simulink model "Model"  (R2016a)
settings: Solver=ode23tb  StartTime=0.0  StopTime=1  RelTol=1e-3
libraries: powerlib_meascontrol x6, powerlib x6
settings Model: Creator=Rodney Tan  LastModifiedBy=Rodney Tan
settings DataIOCC: LimitDataPoints=on  SaveFormat=Array
settings DebuggingCC: SolverPrmCheckMsg=warning
settings HardwareCC: ProdBitPerPointer=32  ProdLargestAtomicFloat=None  ProdIntDivRoundTo=Undefined  ProdEndianess=Unspecified  ProdWordSize=32  ProdHWDeviceType=32-bit Generic
settings ModelReferenceCC: PropagateSignalLabelsOutOfModel=off
settings ConfigComp: CovModelRefEnable=Off  CovSFcnEnable=off

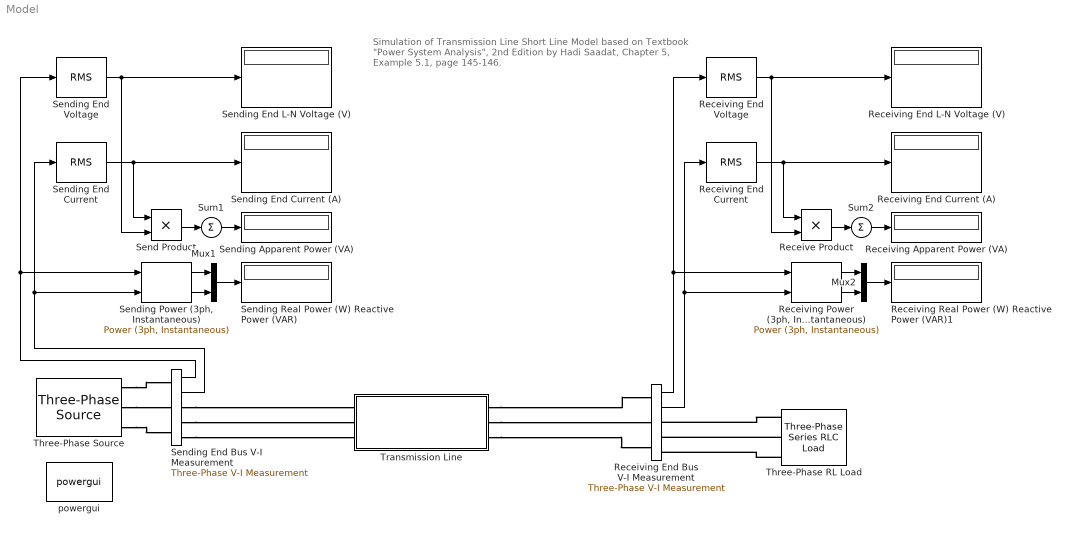
== system Model ==
  note: Simulation of Transmission Line
      | Short Line Model based on Textbook
      | "Power System Analysis", 2nd Edition
      | by Hadi Saadat, Chapter 5, Example 5.1,
      | page 145-146.
  Mux1 : Mux  Inputs=2
  Mux2 : Mux  Inputs=2
  Receive Product : Product
  Receiving Apparent Power (VA) : Display
  Receiving End Current : powerlib_meascontrol/Measurements/RMS  TrueRMS=on  Freq=60  RMSInit=0  Ts=0
  Receiving End Voltage : powerlib_meascontrol/Measurements/RMS  TrueRMS=on  Freq=60  RMSInit=0  Ts=0
  Receiving End Bus V-I Measurement : powerlib/Measurements/Three-Phase V-I Measurement  VoltageMeasurement=phase-to-ground  SetLabelV=off  LabelV=Vabc  Vpu=off  VpuLL=off  CurrentMeasurement=yes  SetLabelI=off  LabelI=Iabc  Ipu=off  Pbase=100e6  Vbase=500e3  OutputType=Complex  PhasorSimulation=off  PSBequivalent=0
  Receiving End Current (A) : Display
  Receiving End L-N Voltage (V) : Display
  "Receiving Power (3ph, Instantaneous)" : powerlib_meascontrol/Measurements/Power (3ph, Instantaneous)
  Receiving Real Power (W) Reactive Power (VAR)1 : Display
  Send Product : Product
  Sending Apparent Power (VA) : Display
  Sending End Current : powerlib_meascontrol/Measurements/RMS  TrueRMS=on  Freq=60  RMSInit=0  Ts=0
  Sending End Voltage : powerlib_meascontrol/Measurements/RMS  TrueRMS=on  Freq=60  RMSInit=0  Ts=0
  Sending End Bus V-I Measurement : powerlib/Measurements/Three-Phase V-I Measurement  VoltageMeasurement=phase-to-ground  SetLabelV=off  LabelV=Vabc  Vpu=off  VpuLL=off  CurrentMeasurement=yes  SetLabelI=off  LabelI=Iabc  Ipu=off  Pbase=100e6  Vbase=500e3  OutputType=Complex  PhasorSimulation=off  PSBequivalent=0
  Sending End Current (A) : Display
  Sending End L-N Voltage (V) : Display
  "Sending Power (3ph, Instantaneous)" : powerlib_meascontrol/Measurements/Power (3ph, Instantaneous)
  Sending Real Power (W) Reactive Power (VAR) : Display
  Sum1 : Sum  Inputs=1
  Sum2 : Sum  Inputs=1
  Three-Phase RL Load : powerlib/Elements/Three-Phase Series RLC Load  LConnTagsString=A|B|C  Configuration=Y (grounded)  NominalVoltage=220e3  Vabc=[1e3 1e3 1e3]  Vabcp=[1e3 1e3 1e3]  NominalFrequency=60  UnbalancedPower=off  ActivePower=304.8e6  InductivePower=228.6e6  CapacitivePower=0  Pabc=[10e3 9e3 11e3]  QLabc=[100 90 110]  QCabc=[100 90 110]  Pabcp=[10e3 9e3 11e3]  QLabcp=[100 90 110]  QCabcp=[100 90 110]  Measurements=None  LoadType=constant Z
  Three-Phase Source : powerlib/Electrical Sources/Three-Phase Source  InternalConnection=Yg  VoltagePhases=off  Voltage=250e3  PhaseAngle=0  Voltage_phases=[25e3 25e3 25e3]/sqrt(3)  PhaseAngles_phases=[0 -120 +120]  Frequency=60  NonIdealSource=off  SpecifyImpedance=off  Resistance=0  Inductance=0  ShortCircuitLevel=100e6  BaseVoltage=250e3  XRratio=7  BusType=swing  Pref=0  Qref=0  Prefabc=[10e3, 10e3, 10e3]  Qrefabc=[0, 0, 0]  Qmin=-inf  Qmax=inf
  Transmission Line : Subsystem  mask(Transmission Line Short Line Model){f=60, LineProperty=Resistance and Inductance, R=0.15, L=0.0013263, Z=0.15+0.5i, Length=40}
      mask prompts: f "Line Frequency (Hz)"; LineProperty "Line Electrical Property in"; R "Resistance Per Unit Length (Ohms/km)"; L "Inductance Per Unit Length (H/km)"; Z "Impedance Per Unit Length (R+Li/km)"; Length "Line Length (km)"
      mask help:
      | Transmission Line Short Line Model developed by Dr Rodney Tan
      | Version 1.0 (Oct 2017)
      |
      | Transmission line short line model block is compute using three phase series RL branch based on its line length (km), resistance per unit length (Ohms/km), inductance per unit length (H/km) or Impedance per unit length (R+Li/km) in complex number.
      mask TypeOptions f: 50 | 60
      mask TypeOptions LineProperty: Resistance and Inductance | Impedance
      mask Callback LineProperty:
      | switch(get_param(gcb,'LineProperty'))
      |     case 'Resistance and Inductance'
      |         set_param(gcb,'MaskEnables',{'on','on','on','on','off','on'});
      |     otherwise
      |         set_param(gcb,'MaskEnables',{'on','on','off','off','on','on'});
      | end
      mask Callback R:
      | R = str2double(get_param(gcb,'R'));
      | L = str2double(get_param(gcb,'L'));
      | f = str2double(get_param(gcb,'f'));
      | set_param(gcb,'Z',num2str(complex(R,2*pi*f*L)));
      mask Callback L:
      | R = str2double(get_param(gcb,'R'));
      | L = str2double(get_param(gcb,'L'));
      | f = str2double(get_param(gcb,'f'));
      | set_param(gcb,'Z',num2str(complex(R,2*pi*f*L)));
      mask Callback Z:
      | Z = str2double(get_param(gcb,'Z'));
      | if ~any(imag(Z))||isnan(Z)
      |     msgbox('Line Impedance must be in Complex Number',...
      |     'Invalid Value !','error');
      |     set_param(gcb,'Z','0.15+0.5i');
      |     return
      | end
      | f = str2double(get_param(gcb,'f'));
      | set_param(gcb,'R',num2str(real(Z)));
      | set_param(gcb,'L',num2str(imag(Z)/(2*pi*f)));
      mask Callback Length:
      | Length = str2double(get_param(gcb,'Length'));
      | if (Length > 100)||(Length < 0.1)||isnan(Length)
      |     msgbox('Line Length must be in the range of 0.1-100',...
      |     'Invalid Value !','error');
      |     set_param(gcb,'Length','40');
      | end
      mask Display:
      | disp('Short Line Model');
      | port_label('lconn',1,'A');
      | port_label('lconn',2,'B');
      | port_label('lconn',3,'C');
      | port_label('rconn',1,'a');
      | port_label('rconn',2,'b');
      | port_label('rconn',3,'c');
  powergui : powerlib/powergui  Priority=1  SimulationMode=Continuous  SolverType=Tustin  SampleTime=50e-6  frequency=60  SPID=off  DisableSnubberDevices=off  DisableRonSwitches=off  DisableVfSwitches=off  SwTol=0  DisplayEquations=off  Interpol=off  ExternalGateDelay=off  methode=off  Ts=0  FunctionMessages=off  echomessages=off  HookPort=off  EnableUseOfTLC=off  x0status=blocks  frequencyindice=60  Pbase=100e6  ErrMax=1e-4  Iterations=50  UnitsV=kV  UnitsW=MW  buscounter=0  RestoreLinks=warning  ResistiveCurrentMeasurement=off  Frange=[0:2:500]  Ylog=off  Xlog=on  ShowGrid=off  save=off  variable=ZData  structure=0  ZoomFFT=off  StartTime=0.0  cycles=1  DisplayStyle=1  fundamental=60  FreqAxis=off  MaxFrequency=1000  frequencyindicesteady=1  RmsSteady=1  display=off
  wires:
  Sending End Bus V-I Measurement/1 -> "Sending Power (3ph, Instantaneous)"/1, Sending End Voltage/1
  Sending End Voltage/1 -> Send Product/2, Sending End L-N Voltage (V)/1
  Sending End Bus V-I Measurement/2 -> "Sending Power (3ph, Instantaneous)"/2, Sending End Current/1
  Sending End Current/1 -> Send Product/1, Sending End Current (A)/1
  "Sending Power (3ph, Instantaneous)"/1 -> Mux1/1
  "Sending Power (3ph, Instantaneous)"/2 -> Mux1/2
  Mux1/1 -> Sending Real Power (W) Reactive Power (VAR)/1
  Send Product/1 -> Sum1/1
  Sum1/1 -> Sending Apparent Power (VA)/1
  Receiving End Bus V-I Measurement/1 -> "Receiving Power (3ph, Instantaneous)"/1, Receiving End Voltage/1
  Receiving End Voltage/1 -> Receive Product/2, Receiving End L-N Voltage (V)/1
  Receiving End Bus V-I Measurement/2 -> "Receiving Power (3ph, Instantaneous)"/2, Receiving End Current/1
  Receiving End Current/1 -> Receive Product/1, Receiving End Current (A)/1
  "Receiving Power (3ph, Instantaneous)"/1 -> Mux2/1
  "Receiving Power (3ph, Instantaneous)"/2 -> Mux2/2
  Mux2/1 -> Receiving Real Power (W) Reactive Power (VAR)1/1
  Receive Product/1 -> Sum2/1
  Sum2/1 -> Receiving Apparent Power (VA)/1
  connections:
  Three-Phase Source/RConn2 -- Sending End Bus V-I Measurement/LConn2
  Three-Phase RL Load/LConn1 -- Receiving End Bus V-I Measurement/RConn1
  Three-Phase RL Load/LConn2 -- Receiving End Bus V-I Measurement/RConn2
  Three-Phase RL Load/LConn3 -- Receiving End Bus V-I Measurement/RConn3
  Three-Phase Source/RConn1 -- Sending End Bus V-I Measurement/LConn1
  Three-Phase Source/RConn3 -- Sending End Bus V-I Measurement/LConn3
  Transmission Line/RConn1 -- Receiving End Bus V-I Measurement/LConn1
  Sending End Bus V-I Measurement/RConn1 -- Transmission Line/LConn1
  Sending End Bus V-I Measurement/RConn2 -- Transmission Line/LConn2
  Transmission Line/RConn2 -- Receiving End Bus V-I Measurement/LConn2
  Sending End Bus V-I Measurement/RConn3 -- Transmission Line/LConn3
  Transmission Line/RConn3 -- Receiving End Bus V-I Measurement/LConn3

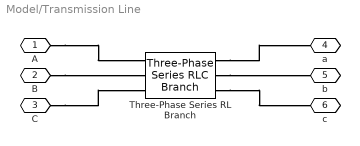
== system Model/Transmission Line ==
  Three-Phase Series RL Branch : powerlib/Elements/Three-Phase Series RLC Branch  LConnTagsString=A|B|C  RConnTagsString=A|B|C  BranchType=RL  Resistance=R*Length  Inductance=L*Length  Capacitance=1e-6  Measurements=None
  A : PMIOPort  Port=1  Side=Left
  B : PMIOPort  Port=2  Side=Left
  C : PMIOPort  Port=3  Side=Left
  a : PMIOPort  Port=4  Side=Right
  b : PMIOPort  Port=5  Side=Right
  c : PMIOPort  Port=6  Side=Right
  connections:
  Three-Phase Series RL Branch/RConn1 -- a/RConn1
  Three-Phase Series RL Branch/RConn3 -- c/RConn1
  A/RConn1 -- Three-Phase Series RL Branch/LConn1
  Three-Phase Series RL Branch/RConn2 -- b/RConn1
  C/RConn1 -- Three-Phase Series RL Branch/LConn3
  B/RConn1 -- Three-Phase Series RL Branch/LConn2
